simulink model "Torque_vectoring_2023a"  (R2023a)
settings: Solver=VariableStepAuto  StartTime=0.0  StopTime=75  RelTol=1e-3
values from neighbouring files (symbols this model uses):
  cf = 615.02    [torque_vectoring_workspace.m]
  cr = 611.27    [torque_vectoring_workspace.m]
  gr = 10.05    [torque_vectoring_workspace.m]
  izz = 47.563    [torque_vectoring_workspace.m]
  lf = 752.15    [torque_vectoring_workspace.m]
  lr = 782.85    [torque_vectoring_workspace.m]
  m = 270    [torque_vectoring_workspace.m]
  rw = 228.6    [torque_vectoring_workspace.m]
  tr = 1150/2    (= 575)    [torque_vectoring_workspace.m]
  vx = 40    [torque_vectoring_workspace.m]
libraries: autolibshared x1, slpidlib x1, simulink x1
settings Model: Creator=Rajdeep  LastModifiedBy=Rajdeep

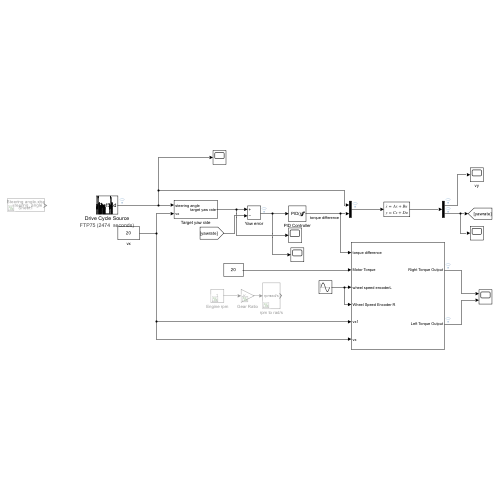
[thumbnail: Simulink's stored preview of the top-level diagram]
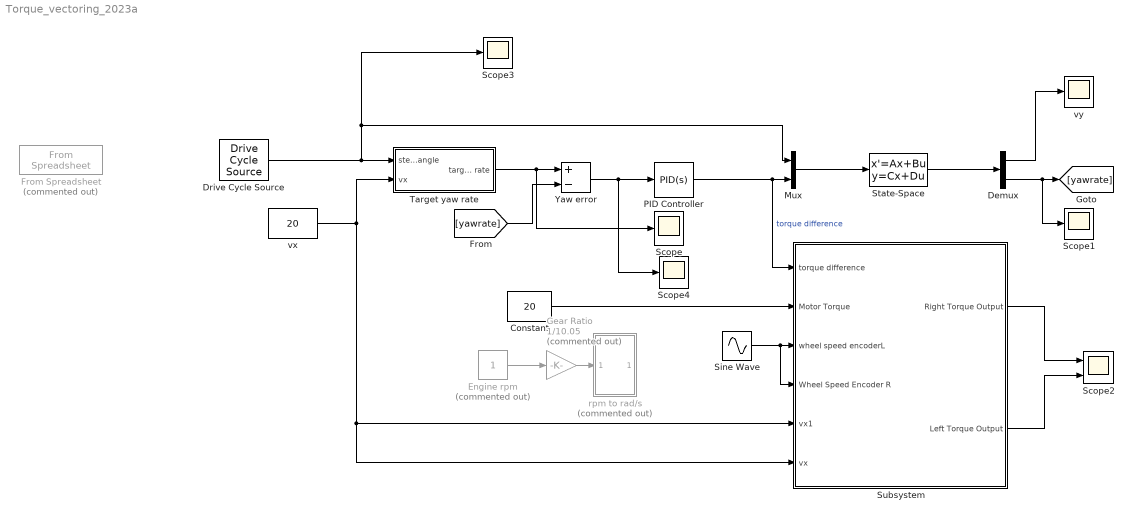
== system Torque_vectoring_2023a ==
  Constant : Constant  Value=20
  Demux : Demux  Outputs=2
  Drive Cycle Source : autolibshared/Drive Cycle Source  cycleVar=FTP75  fileVar=cycleFTP75.mat  tfinal="2474  seconds"  cycleRepeat=off  outAccPort=off  outGearPort=off  gearList=No gear data  t_wot1=5  xdot_woto=0  xdot_wot1=30  t_wot2=20  xdot_wot2=0  t_wotend=30  srcUnit=m/s  outUnit=m/s  srcAccUnit=m/s/s  outAccUnit=m/s^2  dt=0  aMode=1  faultOption=off  velBnd=2  velBndUnit=mph  inUnit=m/s  timeBnd=1  failOption=off  stopSim=off  maxFaultCnt=10  maxFaultTime=2  maxTotFaultTime=15  traceOption=off  dtTrace=1  traceWindow=10  lastDCname=FTP75  lastOutUnit=mph  lastDT=0  lastTB=1  lastSB=2  forceCalcBound=off
  Engine rpm : Constant  Commented=on
  From Spreadsheet : FromSpreadsheet  Commented=on  FileName=Steering angle.xlsx
  Gear Ratio : Gain  Commented=on  Gain=1/10.05
  Mux : Mux  Inputs=2
  PID Controller : slpidlib/PID Controller  Controller=PID  Form=Parallel  TimeDomain=Continuous-time  UseExternalTs=off  SampleTime=-1  IntegratorMethod=Forward Euler  FilterMethod=Forward Euler  ControllerParametersSource=internal  P=-593087.963194818  I=-4076904.53463297  UseKiTs=off  D=-7305.38937374687  N=44.6760543164951  UseFilter=on  TunerSelectOption=Transfer Function Based (PID Tuner App)  InitialConditionSource=internal  InitialConditionForIntegrator=0  InitialConditionForFilter=0  DifferentiatorICPrevScaledInput=0  ExternalReset=none  TrackingMode=off  Kt=1  LimitOutput=on  SatLimitsSource=internal  UpperSaturationLimit=29.2  LowerSaturationLimit=-29.2  LinearizeAsGain=off  AntiWindupMode=clamping  Kb=1  LimitIntegrator=off  UpperIntegratorSaturationLimit=inf  LowerIntegratorSaturationLimit=-inf  POutMin=[]  POutMax=[]  IOutMin=[]  IOutMax=[]  DOutMin=[]  DOutMax=[]  NOutMin=[]  NOutMax=[]  SumOutMin=[]  SumOutMax=[]  SaturationOutMin=[]  SaturationOutMax=[]  PParamMin=[]  PParamMax=[]  IParamMin=[]  IParamMax=[]  DParamMin=[]  DParamMax=[]  NParamMin=[]  NParamMax=[]  KbParamMin=[]  KbParamMax=[]  KtParamMin=[]  KtParamMax=[]  KbOutMin=[]  KbOutMax=[]  KtOutMin=[]  KtOutMax=[]  IntegratorOutMin=[]  IntegratorOutMax=[]  FilterOutMin=[]  FilterOutMax=[]  SumI1OutMin=[]  SumI1OutMax=[]  SumI2OutMin=[]  SumI2OutMax=[]  SumI3OutMin=[]  SumI3OutMax=[]  SumI4OutMin=[]  SumI4OutMax=[]  SumDOutMin=[]  SumDOutMax=[]  DifferentiatorOutMin=[]  DifferentiatorOutMax=[]  FilterDiffOutCoefMin=[]  FilterDiffOutCoefMax=[]  ReciprocalOutMin=[]  ReciprocalOutMax=[]  SumDenOutMin=[]  SumDenOutMax=[]  SumNumOutMin=[]  SumNumOutMax=[]  DivideOutMin=[]  DivideOutMax=[]  UdiffTsProdOutMin=[]  UdiffTsProdOutMax=[]  NTsProdOutMin=[]  NTsProdOutMax=[]  UintegralTsProdOutMin=[]  UintegralTsProdOutMax=[]  UngainTsProdOutMin=[]  UngainTsProdOutMax=[]  ClampingZeroOutDataTypeStr=Inherit: Inherit via back propagation  ClampingZeroOutMin=[]  ClampingZeroOutMax=[]  FilterDenConstantOutDataTypeStr=Inherit: Inherit via back propagation  FilterDenConstantOutMin=[]  FilterDenConstantOutMax=[]  PCopyOutDataTypeStr=Inherit: Inherit via back propagation  PCopyOutMin=[]  PCopyOutMax=[]  NCopyOutDataTypeStr=Inherit: Inherit via back propagation  NCopyOutMin=[]  NCopyOutMax=[]  IntegratorContinuousStateAttributes=''  IntegratorStateMustResolveToSignalObject=off  IntegratorRTWStateStorageClass=Auto  FilterContinuousStateAttributes=''  FilterStateMustResolveToSignalObject=off  FilterRTWStateStorageClass=Auto  ParallelPVariant=InternalParameters  IdealPVariant=Disabled  IVariant=InternalParameters  DVariant=InternalParameters  IntegratorVariant=Continuous  SatVariant=Enabled  AWVariant=ContClampingParallel  PCopyVariant=Disabled  TRVariant=Disabled  FdbkBlocksVariant=Forward  IdealPFdbkVariant=Disabled  SatFdbkVariant=Disabled  DerivativeFilterVariant=ContFilter  NVariant=InternalParameters  NCopyVariant=Disabled  FilterICVariant=InternalICsFilter  IntegratorICVariant=InternalICs  ExternalResetVariant=Disabled  TRSumVariant=Passthrough  SumFdbkVariant=Disabled  SumVariant=Sum_PID  TsampFilterVariant=InternalTs  TsampNgainVariant=Passthrough  TsampIntegralVariant=Disabled_SignalSpec  ExternalSaturationOutDataTypeStr=Inherit: Same as second input
  Scope{,1,3..4} (4 alike) : Scope
  Scope2 : Scope  NumInputPorts=2
  Sine Wave : Sin  Frequency=10  SampleTime=0
  State-Space : StateSpace  A=[-(cf +cr)/(m*vx), (-lf*cf + lr*cr)/(m*vx) - vx ; (-lf*cf + lr*cr)/(izz*vx), -(lf*lf*cf + lr*lr*cr)/(izz*vx)]  B=[ cf/(m*vx), 0 ; lf*cf/izz, 2*tr*gr / (izz*rw) ]  C=[1,0;1,0]  D=[0,0 ; 0,0]  InitialCondition=0
  Subsystem : Subsystem
  Target yaw rate : Subsystem
  Yaw error : Sum  Inputs=+-
  rpm to rad/s : Subsystem  Commented=on
  vx : Constant  Value=20
  vy : Scope
  wires:
  Target yaw rate/1(target yaw rate) -> Scope/1, Yaw error/1
  Yaw error/1 -> Scope4/1, PID Controller/1
  Mux/1 -> State-Space/1
  vx/1 -> Subsystem/6(vx), Subsystem/5(vx1), Target yaw rate/2(vx)
  PID Controller/1 -> Subsystem/1(torque difference), Mux/2  "torque difference"
  State-Space/1 -> Demux/1
  Demux/2 -> [yawrate], Scope1/1
  [yawrate] -> Yaw error/2
  Demux/1 -> vy/1
  Subsystem/1(Right Torque Output) -> Scope2/1
  Subsystem/2(Left Torque Output) -> Scope2/2
  Constant/1 -> Subsystem/2(Motor Torque)
  Engine rpm/1 -> Gear Ratio/1
  Gear Ratio/1 -> rpm to rad/s/1(rpm)
  Drive Cycle Source/1 -> Scope3/1, Mux/1, Target yaw rate/1(steering angle)
  Sine Wave/1 -> Subsystem/4(Wheel Speed Encoder R), Subsystem/3(wheel speed encoderL)

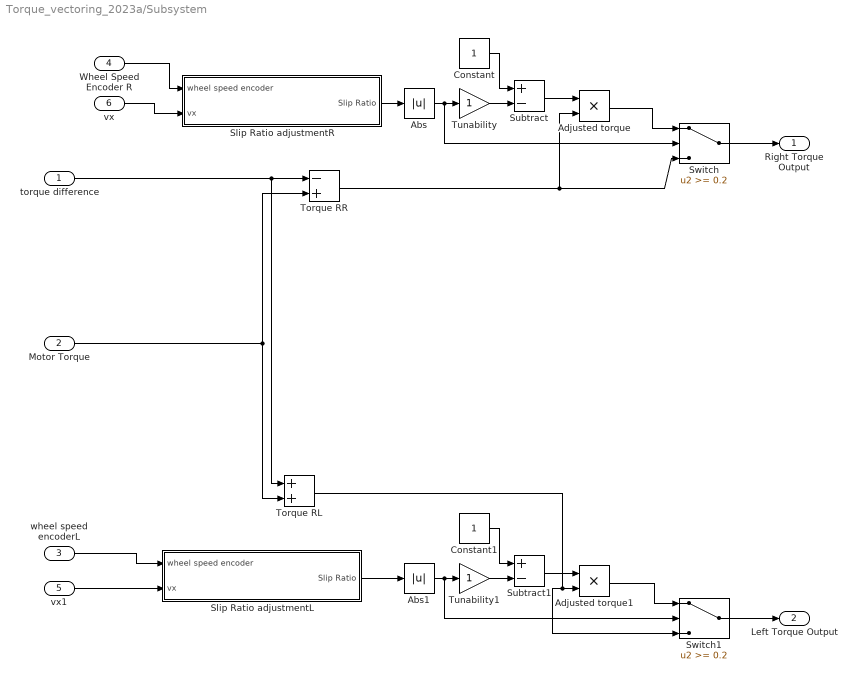
== system Torque_vectoring_2023a/Subsystem ==
  torque difference : Inport
  Motor Torque : Inport  Port=2
  wheel speed encoderL : Inport  Port=3
  Wheel Speed Encoder R : Inport  Port=4
  vx1 : Inport  Port=5
  vx : Inport  Port=6
  Abs : Abs  SaturateOnIntegerOverflow=off
  Abs1 : Abs  SaturateOnIntegerOverflow=off
  Adjusted torque : Product
  Adjusted torque1 : Product
  Constant : Constant
  Constant1 : Constant
  Slip Ratio adjustmentL : Subsystem
  Slip Ratio adjustmentR : Subsystem
  Subtract : Sum  Inputs=+-
  Subtract1 : Sum  Inputs=+-
  Switch : Switch  Threshold=0.2  ZeroCross=off  SaturateOnIntegerOverflow=off  InputSameDT=off
  Switch1 : Switch  Threshold=0.2  ZeroCross=off  SaturateOnIntegerOverflow=off  InputSameDT=off
  Torque RL : Sum
  Torque RR : Sum  Inputs=-+
  Tunability : Gain
  Tunability1 : Gain
  Right Torque Output : Outport
  Left Torque Output : Outport  Port=2
  wires:
  Motor Torque/1 -> Torque RL/2, Torque RR/2
  torque difference/1 -> Torque RL/1, Torque RR/1
  vx1/1 -> Slip Ratio adjustmentL/2(vx)
  wheel speed encoderL/1 -> Slip Ratio adjustmentL/1(wheel speed encoder)
  Wheel Speed Encoder R/1 -> Slip Ratio adjustmentR/1(wheel speed encoder)
  vx/1 -> Slip Ratio adjustmentR/2(vx)
  Tunability/1 -> Subtract/2
  Constant/1 -> Subtract/1
  Subtract/1 -> Adjusted torque/1
  Torque RR/1 -> Switch/3, Adjusted torque/2
  Slip Ratio adjustmentR/1(Slip Ratio) -> Abs/1
  Abs/1 -> Switch/2, Tunability/1
  Adjusted torque/1 -> Switch/1
  Switch/1 -> Right Torque Output/1
  Switch1/1 -> Left Torque Output/1
  Subtract1/1 -> Adjusted torque1/1
  Tunability1/1 -> Subtract1/2
  Adjusted torque1/1 -> Switch1/1
  Abs1/1 -> Switch1/2, Tunability1/1
  Constant1/1 -> Subtract1/1
  Slip Ratio adjustmentL/1(Slip Ratio) -> Abs1/1
  Torque RL/1 -> Switch1/3, Adjusted torque1/2

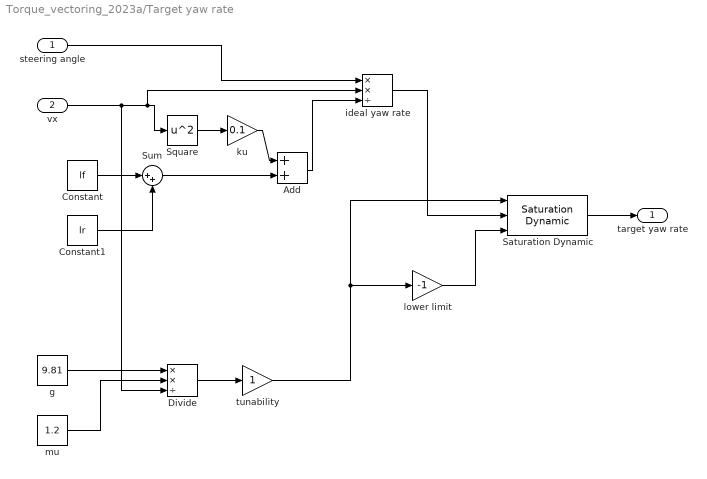
== system Torque_vectoring_2023a/Target yaw rate ==
  steering angle : Inport
  vx : Inport  Port=2
  Add : Sum
  Constant : Constant  Value=lf
  Constant1 : Constant  Value=lr
  Divide : Product  Inputs=**/
  Saturation Dynamic : simulink/Discontinuities/Saturation Dynamic  OutMin=[]  OutMax=[]  OutDataTypeStr=Inherit: Same as second input  OutDataType=fixdt(1, 16)  OutScaling=2^-10  DoSatur=off
  Square : Math  Operator=square
  Sum : Sum  Inputs=|++
  g : Constant  Value=9.81
  ideal yaw rate : Product  Inputs=**/
  ku : Gain  Gain=0.1
  lower limit : Gain  Gain=-1
  mu : Constant  Value=1.2
  tunability : Gain
  target yaw rate : Outport
  wires:
  vx/1 -> ideal yaw rate/2, Square/1, Divide/3
  Constant/1 -> Sum/1
  Constant1/1 -> Sum/2
  Sum/1 -> Add/2
  Square/1 -> ku/1
  ku/1 -> Add/1
  ideal yaw rate/1 -> Saturation Dynamic/2
  Add/1 -> ideal yaw rate/3
  steering angle/1 -> ideal yaw rate/1
  g/1 -> Divide/1
  mu/1 -> Divide/2
  Divide/1 -> tunability/1
  tunability/1 -> lower limit/1, Saturation Dynamic/1
  lower limit/1 -> Saturation Dynamic/3
  Saturation Dynamic/1 -> target yaw rate/1

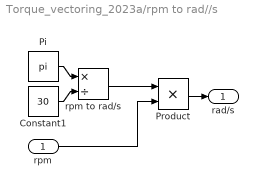
== system Torque_vectoring_2023a/rpm to rad//s ==
  rpm : Inport
  Constant1 : Constant  Value=30
  Pi : Constant  Value=pi  OutDataTypeStr=Inherit: Inherit via back propagation
  Product : Product
  rpm to rad/s : Product  Inputs=*/
  rad/s : Outport
  wires:
  rpm/1 -> Product/2
  Constant1/1 -> rpm to rad/s/2
  Product/1 -> rad/s/1
  Pi/1 -> rpm to rad/s/1
  rpm to rad/s/1 -> Product/1

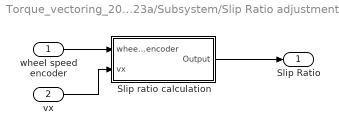
== system Torque_vectoring_2023a/Subsystem/Slip Ratio adjustmentL ==
  wheel speed encoder : Inport
  vx : Inport  Port=2
  Slip ratio calculation : Subsystem
  Slip Ratio : Outport
  wires:
  wheel speed encoder/1 -> Slip ratio calculation/1(wheel speed encoder)
  vx/1 -> Slip ratio calculation/2(vx)
  Slip ratio calculation/1(Output) -> Slip Ratio/1

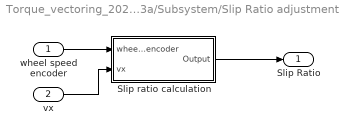
== system Torque_vectoring_2023a/Subsystem/Slip Ratio adjustmentR ==
  wheel speed encoder : Inport
  vx : Inport  Port=2
  Slip ratio calculation : Subsystem
  Slip Ratio : Outport
  wires:
  wheel speed encoder/1 -> Slip ratio calculation/1(wheel speed encoder)
  vx/1 -> Slip ratio calculation/2(vx)
  Slip ratio calculation/1(Output) -> Slip Ratio/1

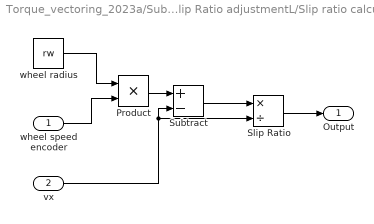
== system Torque_vectoring_2023a/Subsystem/Slip Ratio adjustmentL/Slip ratio calculation ==
  wheel speed encoder : Inport
  vx : Inport  Port=2
  Product : Product
  Slip Ratio : Product  Inputs=*/
  Subtract : Sum  Inputs=+-
  wheel radius : Constant  Value=rw
  Output : Outport
  wires:
  wheel radius/1 -> Product/1
  wheel speed encoder/1 -> Product/2
  Product/1 -> Subtract/1
  vx/1 -> Subtract/2, Slip Ratio/2
  Subtract/1 -> Slip Ratio/1
  Slip Ratio/1 -> Output/1

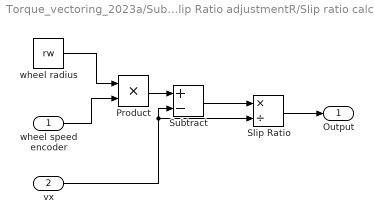
== system Torque_vectoring_2023a/Subsystem/Slip Ratio adjustmentR/Slip ratio calculation ==
  wheel speed encoder : Inport
  vx : Inport  Port=2
  Product : Product
  Slip Ratio : Product  Inputs=*/
  Subtract : Sum  Inputs=+-
  wheel radius : Constant  Value=rw
  Output : Outport
  wires:
  wheel radius/1 -> Product/1
  wheel speed encoder/1 -> Product/2
  Product/1 -> Subtract/1
  vx/1 -> Subtract/2, Slip Ratio/2
  Subtract/1 -> Slip Ratio/1
  Slip Ratio/1 -> Output/1
